simulink model "example12"  (R2024b)
settings: Solver=VariableStepAuto  StartTime=0.0  StopTime=12  RelTol=1e-3
values from neighbouring files (symbols this model uses):
  A = [-a_(2:end)', [1; 0]]    [example1_2.m]    (also in example1_22.m)
  a = [1, -0.8]    [example1_2.m]    (also in example1_22.m)
  B = b(2:3)'    [example1_2.m]    (also in example1_22.m)
  b = [0, 0.4, 0.6]    [example1_2.m]    (also in example1_22.m)
  D = -a_(2:end)'    [example1_2.m]    (also in example1_22.m)
  delta = [1, -1]    [example1_2.m]    (also in example1_22.m)
  H = [1, 0]    [example1_2.m]    (also in example1_22.m)
  KE = K*E    [example1_2.m]    (also in example1_22.m)
  KF = K*F    [example1_2.m]    (also in example1_22.m)
  Kr = sum(K)    [example1_2.m]    (also in example1_22.m)
undefined symbols (not defined in the file or in its folder): dspblkCoreblockFVToolHelper, gcbh
settings Model: Creator=room2  LastModifiedBy=room2

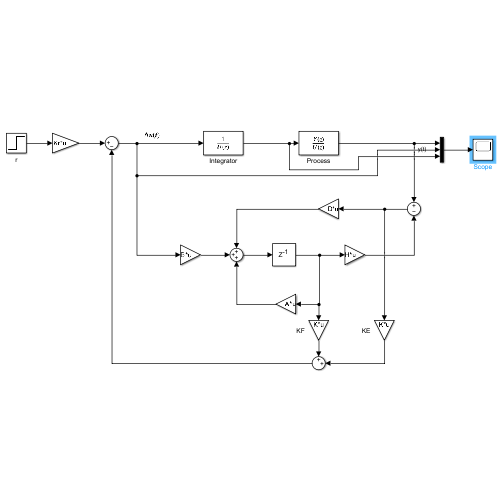
[thumbnail: Simulink's stored preview of the top-level diagram]
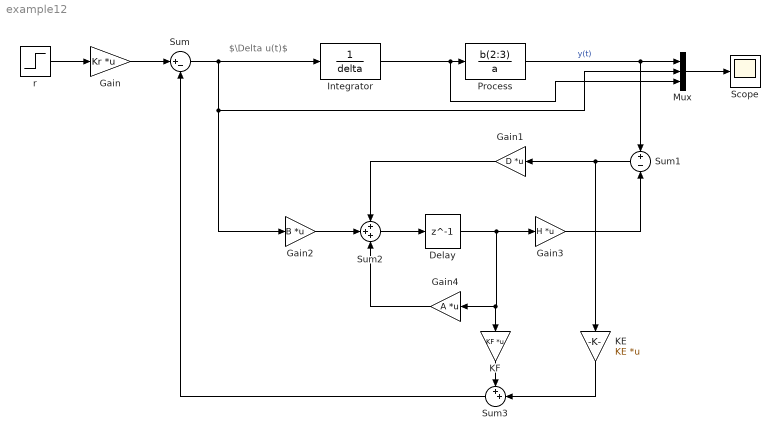
== system example12 ==
  note: $\Delta u(t)$
  Delay : Delay  DelayLength=1
  Gain : Gain  Gain=Kr  Multiplication=Matrix(K*u)
  Gain1 : Gain  Gain=D  Multiplication=Matrix(K*u)
  Gain2 : Gain  Gain=B  Multiplication=Matrix(K*u)
  Gain3 : Gain  Gain=H  Multiplication=Matrix(K*u)
  Gain4 : Gain  Gain=A  Multiplication=Matrix(K*u)
  Integrator : DiscreteTransferFcn  LoadFcn=dspblkCoreblockFVToolHelper(gcbh,'load');  Denominator=delta
      settings: CopyFcn=dspblkCoreblockFVToolHelper(gcbh,'copy');  DeleteFcn=dspblkCoreblockFVToolHelper(gcbh,'close');  ModelCloseFcn=dspblkCoreblockFVToolHelper(gcbh,'close');  PreSaveFcn=dspblkCoreblockFVToolHelper(gcbh,'presave');  PostSaveFcn=dspblkCoreblockFVToolHelper(gcbh,'postsave');  CloseFcn=dspblkCoreblockFVToolHelper(gcbh,'close');
  KE : Gain  Gain=KE  Multiplication=Matrix(K*u)
  KF : Gain  Gain=KF  Multiplication=Matrix(K*u)
  Mux : Mux  Inputs=3
  Process : DiscreteTransferFcn  LoadFcn=dspblkCoreblockFVToolHelper(gcbh,'load');  Numerator=b(2:3)  Denominator=a
      settings: CopyFcn=dspblkCoreblockFVToolHelper(gcbh,'copy');  DeleteFcn=dspblkCoreblockFVToolHelper(gcbh,'close');  ModelCloseFcn=dspblkCoreblockFVToolHelper(gcbh,'close');  PreSaveFcn=dspblkCoreblockFVToolHelper(gcbh,'presave');  PostSaveFcn=dspblkCoreblockFVToolHelper(gcbh,'postsave');  CloseFcn=dspblkCoreblockFVToolHelper(gcbh,'close');
  Scope : Scope
  Sum : Sum  Inputs=|+-
  Sum1 : Sum  Inputs=+|-
  Sum2 : Sum  Inputs=+++
  Sum3 : Sum  Inputs=++|
  r : Step  Time=0  SampleTime=0
  wires:
  r/1 -> Gain/1
  Gain/1 -> Sum/1
  Sum/1 -> Mux/2, Gain2/1, Integrator/1
  Integrator/1 -> Mux/3, Process/1
  Sum1/1 -> Gain1/1, KE/1
  Gain1/1 -> Sum2/1
  Sum2/1 -> Delay/1
  Delay/1 -> KF/1, Gain4/1, Gain3/1
  Gain3/1 -> Sum1/2
  Gain4/1 -> Sum2/3
  KF/1 -> Sum3/1
  KE/1 -> Sum3/2
  Gain2/1 -> Sum2/2
  Sum3/1 -> Sum/2
  Process/1 -> Mux/1, Sum1/1  "y(t)"
  Mux/1 -> Scope/1
